simulink model "SHE_simulink"  (R2017a)
settings: Solver=VariableStepDiscrete  StartTime=0.0  StopTime=10  MaxStep=1e-4  RelTol=1e-3  AbsTol=1e-3  EnableMultiTasking=on
values from neighbouring files (symbols this model uses):
  delay_p_n_1 = (theta_1 * T )/ 360 + T/2    [SHE.m]
  delay_p_n_2 = (theta_3 * T) / 360 + T/2    [SHE.m]
  delay_p_n_3 = ((180 - theta_2) * T) / 360 + T/2    [SHE.m]
  delay_p_p_1 = theta_1 * T / 360    [SHE.m]
  delay_p_p_2 = theta_3 * T / 360    [SHE.m]
  delay_p_p_3 = ((180 - theta_2) * T) / 360    [SHE.m]
  period = T    (= 1)    [SHE.m]
  puls_w_n_1 = ((theta_2 - theta_1)*T)/3.6    [SHE.m]
  puls_w_n_2 = 2*((90 - theta_3)*T)/3.6    [SHE.m]
  puls_w_n_3 = ((theta_2 - theta_1)*T)/3.6    [SHE.m]
  puls_w_p_1 = ((theta_2 - theta_1)*T)/3.6    [SHE.m]
  puls_w_p_2 = 2*((90 - theta_3)*T)/3.6    [SHE.m]
  puls_w_p_3 = ((theta_2 - theta_1)*T)/3.6    [SHE.m]
libraries: powerlib x7
settings Model: Creator=mohammad  LastModifiedBy=mohammad
settings DataIOCC: LimitDataPoints=on
settings OptimizationCC: LifeSpan=inf
settings DebuggingCC: AllowSymbolicDim=off  SFUnexpectedBacktrackingDiag=warning  SFNoUnconditionalDefaultTransitionDiag=warning  SFExecutionAtInitializationDiag=none
settings GRTTargetCC: TargetLangStandard=C89/C90 (ANSI)  GeneratePreprocessorConditionals=Disable all
settings ConfigComp: CovMetricSettings=dw  CovHtmlReporting=on  CovSaveCumulativeToWorkspaceVar=on  CovSaveSingleToWorkspaceVar=on  CovExternalEMLEnable=off  CovSFcnEnable=off
settings SimscapeCC: SimscapeLogType=all  SimscapeLogDataHistory=10000

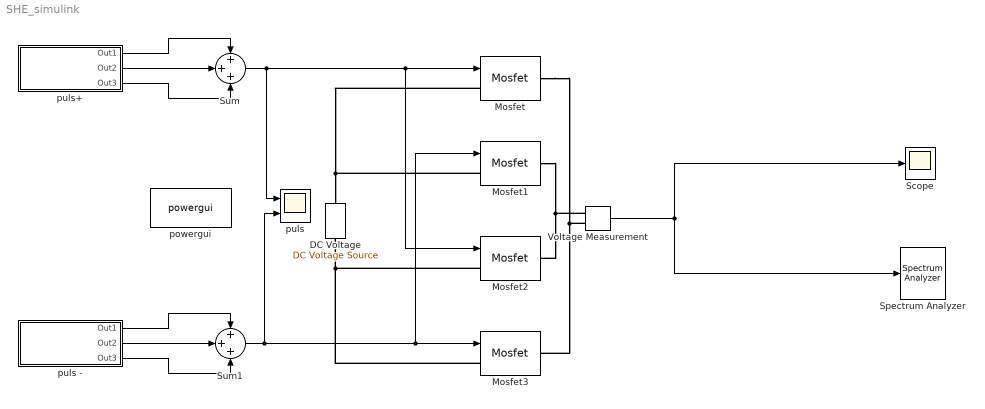
== system SHE_simulink ==
  "DC Voltage " : powerlib/Electrical Sources/DC Voltage Source  Amplitude=100  Measurements=None
  Mosfet{,1..3} (4 alike) : powerlib/Power Electronics/Mosfet  Ron=0.001  Lon=0  Rd=0.01  Vfd=0  IC=0  Rs=1e5  Cs=inf  Measurements=off
  Scope : Scope
  Spectrum Analyzer : SpectrumAnalyzer
  Sum : Sum  Inputs=+++
  Sum1 : Sum  Inputs=+++
  Voltage Measurement : powerlib/Measurements/Voltage Measurement  PhasorSimulation=off  OutputType=Complex  PSBequivalent=0
  powergui : powerlib/powergui  Priority=1  SimulationMode=Discrete  SampleTime=.002  frequency=60  Iterations=50  frequencyindice=0  Pbase=100e6  ErrMax=1e-4  UnitsV=kV  UnitsW=MW  buscounter=0  FunctionMessages=off  echomessages=off  EnableUseOfTLC=off  CurrentSourceSwitches=off  DisableSnubberDevices=off  DisableRonSwitches=off  DisableVfSwitches=off  DisplayEquations=off  SolverType=Tustin/Backward Euler (TBE)  Interpol=off  ExternalGateDelay=off  methode=off  Ts=100  x0status=blocks  SPID=on  SwTol=0  HookPort=off  RestoreLinks=warning  ResistiveCurrentMeasurement=off  Frange=[0:2:500]  Ylog=off  Xlog=on  ShowGrid=off  save=off  variable=ZData  structure=0  ZoomFFT=off  StartTime=0.0  cycles=1  DisplayStyle=1  fundamental=60  FreqAxis=off  MaxFrequency=1000  frequencyindicesteady=1  RmsSteady=1  display=off
  puls : Scope  NumInputPorts=2
  puls - : Subsystem
  puls+ : Subsystem
  wires:
  Sum/1 -> puls/1, Mosfet2/1, Mosfet/1
  Sum1/1 -> puls/2, Mosfet1/1, Mosfet3/1
  puls -/2(Out2) -> Sum1/2
  puls -/1(Out1) -> Sum1/1
  puls -/3(Out3) -> Sum1/3
  puls+/2(Out2) -> Sum/2
  puls+/1(Out1) -> Sum/1
  puls+/3(Out3) -> Sum/3
  Voltage Measurement/1 -> Spectrum Analyzer/1, Scope/1
  connections:
  Mosfet2/LConn1 -- Mosfet3/LConn1 -- "DC Voltage "/LConn1
  Mosfet1/LConn1 -- "DC Voltage "/RConn1 -- Mosfet/LConn1
  Mosfet1/RConn1 -- Mosfet2/RConn1 -- Voltage Measurement/LConn1
  Mosfet/RConn1 -- Mosfet3/RConn1 -- Voltage Measurement/LConn2

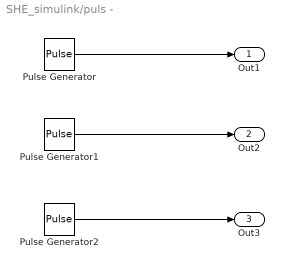
== system SHE_simulink/puls - ==
  Pulse Generator : DiscretePulseGenerator  PulseType=Time based  Period=period  PulseWidth=puls_w_n_1  PhaseDelay=delay_p_n_1
  Pulse Generator1 : DiscretePulseGenerator  PulseType=Time based  Period=period  PulseWidth=puls_w_n_2  PhaseDelay=delay_p_n_2
  Pulse Generator2 : DiscretePulseGenerator  PulseType=Time based  Period=period  PulseWidth=puls_w_n_3  PhaseDelay=delay_p_n_3
  Out1 : Outport
  Out2 : Outport  Port=2
  Out3 : Outport  Port=3
  wires:
  Pulse Generator/1 -> Out1/1
  Pulse Generator1/1 -> Out2/1
  Pulse Generator2/1 -> Out3/1

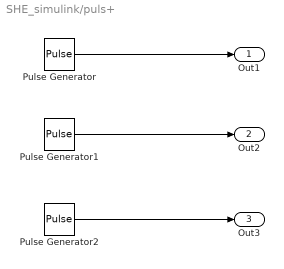
== system SHE_simulink/puls+ ==
  Pulse Generator : DiscretePulseGenerator  PulseType=Time based  Period=period  PulseWidth=puls_w_p_1  PhaseDelay=delay_p_p_1
  Pulse Generator1 : DiscretePulseGenerator  PulseType=Time based  Period=period  PulseWidth=puls_w_p_2  PhaseDelay=delay_p_p_2
  Pulse Generator2 : DiscretePulseGenerator  PulseType=Time based  Period=period  PulseWidth=puls_w_p_3  PhaseDelay=delay_p_p_3
  Out1 : Outport
  Out2 : Outport  Port=2
  Out3 : Outport  Port=3
  wires:
  Pulse Generator/1 -> Out1/1
  Pulse Generator1/1 -> Out2/1
  Pulse Generator2/1 -> Out3/1
